simulink library "TemperatureBlock"  (R2021a)
settings: Solver=ode45  StartTime=0.0  StopTime=10.0  RelTol=1e-3  EnableMultiTasking=on
undefined symbols (not defined in the file): Cj, Cs, Rj, Ru
Description:
  | Thomas Modules
settings Model: Creator=jwchapm2  LastModifiedBy=sfaulk
settings SolverCC: AlgebraicLoopSolver=TrustRegion
settings DataIOCC: LimitDataPoints=on  SaveFormat=Array  ReturnWorkspaceOutputs=off
settings OptimizationCC: ExpressionDepthLimit=2147483647  LifeSpan=inf
settings DebuggingCC: UnderspecifiedInitializationDetection=Classic  MergeDetectMultiDrivingBlocksExec=none  SolverPrmCheckMsg=warning  StateNameClashWarn=warning  SFUnexpectedBacktrackingDiag=warning  SFNoUnconditionalDefaultTransitionDiag=warning  SFExecutionAtInitializationDiag=none  SFMachineParentedDataDiag=warning  ArithmeticOperatorsInVariantConditions=warning
settings HardwareCC: ProdBitPerPointer=32  ProdBitPerSizeT=32  ProdBitPerPtrDiffT=32  ProdLargestAtomicFloat=None  ProdIntDivRoundTo=Undefined  ProdEndianess=Unspecified  ProdWordSize=32  ProdHWDeviceType=32-bit Generic
settings ModelReferenceCC: PropagateSignalLabelsOutOfModel=off
settings SFSimCC: SimUseLocalCustomCode=off  CustomCodeUndefinedFunction=UseInterfaceOnly
settings RTWCC: RTWUseLocalCustomCode=off
settings CodeAppCC: StateflowObjectComments=on
settings GRTTargetCC: TargetLangStandard=C89/C90 (ANSI)
settings ConfigComp: CovMetricSettings=dw  CovSaveCumulativeToWorkspaceVar=on  CovSaveSingleToWorkspaceVar=on  CovExternalEMLEnable=off

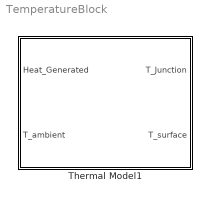
== system TemperatureBlock ==
  Thermal Model1 : Subsystem  mask{Tj_0_M=25, Ts_0_M=25, Cj_M=Cj, Rj_M=Rj, Ru_M=Ru, Cs_M=Cs}
      mask prompts: Tj_0_M "Initial Junction Temperature (°Ra)"; Ts_0_M "Initial Surface Temperature (°Ra)"; Cj_M "Lumped Heat Capacity at Junction (J/°Ra)"; Rj_M "Conduction Resistance b/w Junction and Surface (°Ra/W)"; Ru_M "Convection Resistance b/w Surface and Cooling Flow (°F/W)"; Cs_M "Lumped Heat Capacity at Surface (J/°Ra)"
      mask init:
      | %Get current block name:
      | block = gcb;
      | %{
      | %Blocks under the mask(T_in inport and outport):
      | block2 = [block '/T_ambient'];
      | block3 = [block '/unitsOut'];
      | 
      | %Set T_in unit parameter to correct unit.
      | switch TempIn
      |     case 1 
      |         set_param(block2,'Unit','degF');
      |     case 2
      |         set_param(block2,'Unit','degC');
      |     case 3
      |         set_param(block2,'Unit','degR');
      |     case 4
      |         set_param(block2,'Unit','K');
      | end
      | switch TempOut
      |     case 1 
      |         set_param(block3,'Unit','degF');
      |     case 2
      |         set_param(block3,'Unit','degC');
      |     case 3
      |         set_param(block3,'Unit','degR');
      |     case 4
      |         set_param(block3,'Unit','K');
      | end
      | %}
      mask DialogControl Container7 Prompt: Parameters
      mask Display:
      | %{
      | switch TempIn
      |     case 1
      |         port_label('input', 2, sprintf('T_ambient\n     (%cF)', char(176)));
      |     case 2
      |         port_label('input', 2, sprintf('T_ambient\n     (%cC)', char(176)));
      |     case 3
      |         port_label('input', 2, sprintf('T_ambient\n     (%cRa)', char(176)'));
      |     case 4
      |         port_label('input', 2, sprintf('T_ambient\n     (%cK)', char(176)));
      | end
      | switch TempOut
      |     case 1
      |         port_label('output', 1, sprintf('T_Junction\n   (%cF)', char(176)));
      |         port_label('output', 2, sprintf('T_Surface\n   (%cF)', char(176)));
      |     case 2
      |         port_label('output', 1, sprintf('T_Junction\n   (%cC)', char(176)));
      |         port_label('output', 2, sprintf('T_Surface\n   (%cC)', char(176)));
      |     case 3
      |         port_label('output', 1, sprintf('T_Junction\n   (%cRa)', char(176)));
      |         port_label('output', 2, sprintf('T_Surface\n   (%cRa)', char(176)));
      |     case 4
      |         port_label('output', 1, sprintf('T_Junction\n   (%cK)', char(176)));
      |         port_label('output', 2, sprintf('T_Surface\n   (%cK)', char(176)));
      | end
      | %}
      | port_label('input', 1, 'Heat_Generated (W)');
      | port_label('input', 2, sprintf('T_ambient\n     (%cRa)', char(176)'));
      | port_label('output', 1, sprintf('T_Junction\n   (%cRa)', char(176)));
      | port_label('output', 2, sprintf('T_Surface\n   (%cRa)', char(176)));

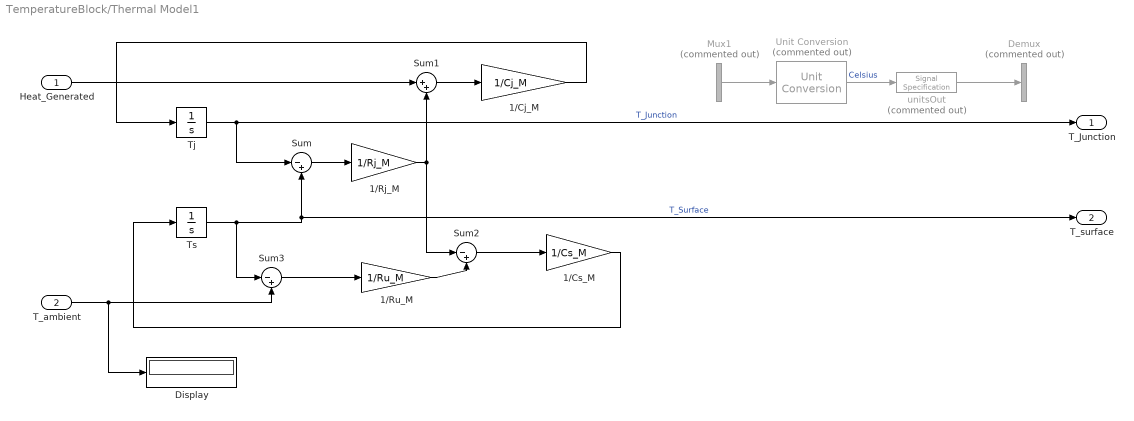
== system TemperatureBlock/Thermal Model1 ==
  Heat_Generated : Inport
  T_ambient : Inport  Port=2  Unit=degR
  1/Cj_M : Gain  Gain=1/Cj_M
  1/Cs_M : Gain  Gain=1/Cs_M
  1/Rj_M : Gain  Gain=1/Rj_M
  1/Ru_M : Gain  Gain=1/Ru_M
  Demux : Demux  Commented=on  Outputs=2
  Display : Display
  Mux1 : Mux  Commented=on  Inputs=2
  Sum : Sum  Inputs=|-+
  Sum1 : Sum  Inputs=|++
  Sum2 : Sum  Inputs=|-+
  Sum3 : Sum  Inputs=|-+
  Tj : Integrator  InitialCondition=Tj_0_M
  Ts : Integrator  InitialCondition=Ts_0_M
  Unit Conversion : UnitConversion  Commented=on
  unitsOut : SignalSpecification  Commented=on  Unit=degR
  T_Junction : Outport  VectorParamsAs1DForOutWhenUnconnected=off
  T_surface : Outport  Port=2  VectorParamsAs1DForOutWhenUnconnected=off
  wires:
  1/Ru_M/1 -> Sum2/2
  Sum3/1 -> 1/Ru_M/1
  1/Cs_M/1 -> Ts/1
  Sum2/1 -> 1/Cs_M/1
  1/Cj_M/1 -> Tj/1
  Sum1/1 -> 1/Cj_M/1
  1/Rj_M/1 -> Sum1/2, Sum2/1
  Sum/1 -> 1/Rj_M/1
  Heat_Generated/1 -> Sum1/1
  T_ambient/1 -> Display/1, Sum3/2
  unitsOut/1 -> Demux/1
  Unit Conversion/1 -> unitsOut/1  "Celsius"
  Mux1/1 -> Unit Conversion/1
  Tj/1 -> T_Junction/1, Sum/1  "T_Junction"
  Ts/1 -> Sum/2, T_surface/1, Sum3/1  "T_Surface"
